simulink model "PID_track"  (R2024b)
settings: Solver=VariableStepAuto  StartTime=0.0  StopTime=t_sim  RelTol=1e-3
values from neighbouring files (symbols this model uses):
  Ax = [0 1; 0 0]    [Main_PID_track.m]
  Ay = [0 1; 0 0]    [Main_PID_track.m]
  b = 0.0245    [Main_PID_track.m]
  Bx = [0 Cx]'    [Main_PID_track.m]
  By = [0 Cy]'    [Main_PID_track.m]
  Cx = m*g*b/(m+J/r^2)/lx    (= 0.943269230769)    [Main_PID_track.m]
  Cy = m*g*b/(m+J/r^2)/ly    (= 1.1445)    [Main_PID_track.m]
  data_sys = [m r g J b lx ly]    [Main_PID_track.m]
  Kb_x = 0.8    [Main_PID_track.m]
  Kb_y = 0.8    [Main_PID_track.m]
  Kd_x = 3    [Main_PID_track.m]
  Kd_y = Kd_x/1.2    (= 2.5)    [Main_PID_track.m]
  Ki_x = 1.5    [Main_PID_track.m]
  Ki_y = Ki_x/1.2    (= 1.25)    [Main_PID_track.m]
  Kp_x = 5    [Main_PID_track.m]
  Kp_y = Kp_x/1.2    (= 4.16666666667)    [Main_PID_track.m]
  lx = 0.182    [Main_PID_track.m]
  ly = 0.150    (= 0.15)    [Main_PID_track.m]
  N_x = 15    [Main_PID_track.m]
  N_y = 15    [Main_PID_track.m]
  ux_lim = 45    [Main_PID_track.m]
  uy_lim = 45    [Main_PID_track.m]
  zx0 = [x0 xp0]'    [Main_PID_track.m]
  zy0 = [y0 yp0]'    [Main_PID_track.m]
undefined symbols (not defined in the file or in its folder): Dx, Dy
libraries: slpidlib x2, simulink x1
settings Model: Creator=nicvi  LastModifiedBy=nicvi

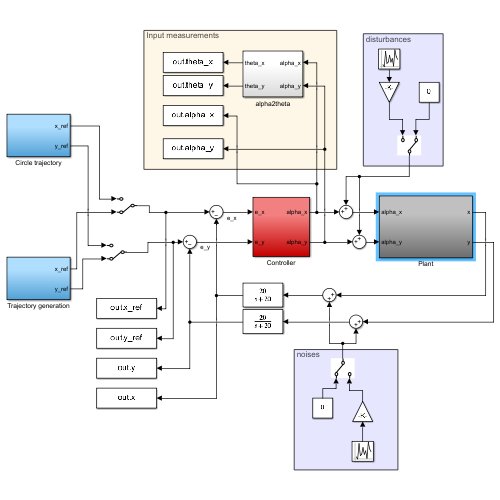
[thumbnail: Simulink's stored preview of the top-level diagram]
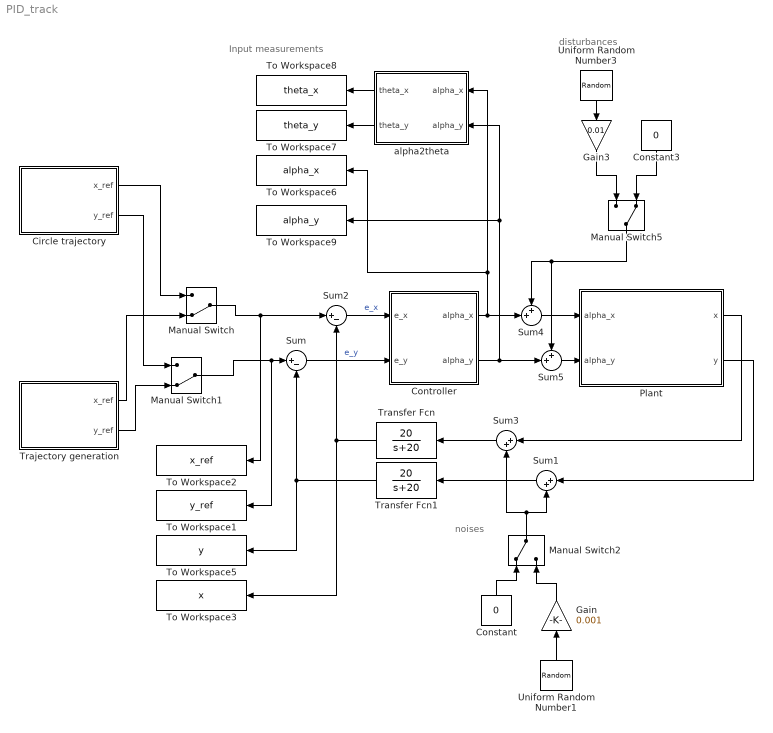
== system PID_track ==
  note: noises
  note: Input measurements
  note: disturbances
  Circle trajectory : Subsystem
  Constant : Constant  Value=0
  Constant3 : Constant  Value=0
  Controller : Subsystem
  Gain : Gain  Gain=0.001
  Gain3 : Gain  Gain=0.01
  Manual Switch : ManualSwitch  CurrentSetting=0
  Manual Switch1 : ManualSwitch  CurrentSetting=0
  Manual Switch2 : ManualSwitch
  Manual Switch5 : ManualSwitch  CurrentSetting=0
  Plant : Subsystem
  Sum : Sum  Inputs=|+-
  Sum1 : Sum  Inputs=|++
  Sum2 : Sum  Inputs=|+-
  Sum3 : Sum  Inputs=|++
  Sum4 : Sum  Inputs=++|
  Sum5 : Sum  Inputs=++|
  To Workspace1 : ToWorkspace  VariableName=y_ref  SampleTime=-1
      settings: Save2DSignal=2-D array (concatenate along first dimension)
  To Workspace2 : ToWorkspace  VariableName=x_ref  SampleTime=-1
      settings: Save2DSignal=2-D array (concatenate along first dimension)
  To Workspace3 : ToWorkspace  VariableName=x  SampleTime=-1
      settings: Save2DSignal=2-D array (concatenate along first dimension)
  To Workspace5 : ToWorkspace  VariableName=y  SampleTime=-1
      settings: Save2DSignal=2-D array (concatenate along first dimension)
  To Workspace6 : ToWorkspace  VariableName=alpha_x  SampleTime=-1
      settings: Save2DSignal=2-D array (concatenate along first dimension)
  To Workspace7 : ToWorkspace  VariableName=theta_y  SampleTime=-1
      settings: Save2DSignal=2-D array (concatenate along first dimension)
  To Workspace8 : ToWorkspace  VariableName=theta_x  SampleTime=-1
      settings: Save2DSignal=2-D array (concatenate along first dimension)
  To Workspace9 : ToWorkspace  VariableName=alpha_y  SampleTime=-1
      settings: Save2DSignal=2-D array (concatenate along first dimension)
  Trajectory generation : Subsystem
  Transfer Fcn : TransferFcn  Numerator=[20]  Denominator=[1 20]
  Transfer Fcn1 : TransferFcn  Numerator=[20]  Denominator=[1 20]
  Uniform Random Number1 : UniformRandomNumber  SampleTime=0.1
  Uniform Random Number3 : UniformRandomNumber  Minimum=5  Maximum=7  SampleTime=0.01
  alpha2theta : Subsystem
  wires:
  Sum2/1 -> Controller/1(e_x)  "e_x"
  Sum/1 -> Controller/2(e_y)  "e_y"
  Controller/1(alpha_x) -> alpha2theta/1(alpha_x), To Workspace6/1, Sum4/2
  Controller/2(alpha_y) -> Sum5/2, alpha2theta/2(alpha_y), To Workspace9/1
  alpha2theta/1(theta_x) -> To Workspace8/1
  alpha2theta/2(theta_y) -> To Workspace7/1
  Plant/2(y) -> Sum1/1
  Plant/1(x) -> Sum3/1
  Circle trajectory/1(x_ref) -> Manual Switch/1
  Manual Switch/1 -> Sum2/1, To Workspace2/1
  Manual Switch1/1 -> To Workspace1/1, Sum/1
  Circle trajectory/2(y_ref) -> Manual Switch1/1
  Trajectory generation/1(x_ref) -> Manual Switch/2
  Trajectory generation/2(y_ref) -> Manual Switch1/2
  Sum1/1 -> Transfer Fcn1/1
  Sum3/1 -> Transfer Fcn/1
  Gain/1 -> Manual Switch2/2
  Manual Switch2/1 -> Sum1/2, Sum3/2
  Uniform Random Number1/1 -> Gain/1
  Transfer Fcn/1 -> Sum2/2, To Workspace3/1
  Transfer Fcn1/1 -> Sum/2, To Workspace5/1
  Constant/1 -> Manual Switch2/1
  Manual Switch5/1 -> Sum4/1, Sum5/1
  Constant3/1 -> Manual Switch5/2
  Uniform Random Number3/1 -> Gain3/1
  Gain3/1 -> Manual Switch5/1
  Sum4/1 -> Plant/1(alpha_x)
  Sum5/1 -> Plant/2(alpha_y)

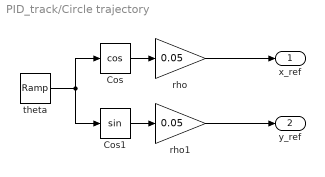
== system PID_track/Circle trajectory ==
  Cos : Trigonometry  Operator=cos
  Cos1 : Trigonometry
  rho : Gain  Gain=0.05
  rho1 : Gain  Gain=0.05
  theta : simulink/Sources/Ramp  slope=2*pi/10  start=0  InitialOutput=0
  x_ref : Outport
  y_ref : Outport  Port=2
  wires:
  theta/1 -> Cos1/1, Cos/1
  Cos/1 -> rho/1
  Cos1/1 -> rho1/1
  rho1/1 -> y_ref/1
  rho/1 -> x_ref/1

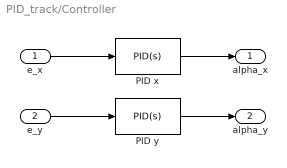
== system PID_track/Controller ==
  e_x : Inport
  e_y : Inport  Port=2
  PID x : slpidlib/PID Controller  Controller=PID  Form=Parallel  TimeDomain=Continuous-time  UseExternalTs=off  SampleTime=-1  IntegratorMethod=Forward Euler  FilterMethod=Forward Euler  ControllerParametersSource=internal  P=Kp_x  I=Ki_x  UseKiTs=off  D=Kd_x  UseExternalDerivativeSource=off  N=N_x  UseFilter=on  TunerSelectOption=Transfer Function Based (PID Tuner App)  InitialConditionSource=internal  InitialConditionForIntegrator=0  InitialConditionForFilter=0  DifferentiatorICPrevScaledInput=0  ExternalReset=none  TrackingMode=off  Kt=1  LimitOutput=on  SatLimitsSource=internal  UpperSaturationLimit=deg2rad(ux_lim)  LowerSaturationLimit=deg2rad(-ux_lim)  LinearizeAsGain=on  AntiWindupMode=back-calculation  Kb=Kb_x  LimitIntegrator=off  UpperIntegratorSaturationLimit=inf  LowerIntegratorSaturationLimit=-inf  POutMin=[]  POutMax=[]  IOutMin=[]  IOutMax=[]  DOutMin=[]  DOutMax=[]  NOutMin=[]  NOutMax=[]  SumOutMin=[]  SumOutMax=[]  SaturationOutMin=[]  SaturationOutMax=[]  PParamMin=[]  PParamMax=[]  IParamMin=[]  IParamMax=[]  DParamMin=[]  DParamMax=[]  NParamMin=[]  NParamMax=[]  KbParamMin=[]  KbParamMax=[]  KtParamMin=[]  KtParamMax=[]  KbOutMin=[]  KbOutMax=[]  KtOutMin=[]  KtOutMax=[]  IntegratorOutMin=[]  IntegratorOutMax=[]  FilterOutMin=[]  FilterOutMax=[]  SumI1OutMin=[]  SumI1OutMax=[]  SumI2OutMin=[]  SumI2OutMax=[]  SumI3OutMin=[]  SumI3OutMax=[]  SumI4OutMin=[]  SumI4OutMax=[]  SumDOutMin=[]  SumDOutMax=[]  DifferentiatorOutMin=[]  DifferentiatorOutMax=[]  FilterDiffOutCoefMin=[]  FilterDiffOutCoefMax=[]  ReciprocalOutMin=[]  ReciprocalOutMax=[]  SumDenOutMin=[]  SumDenOutMax=[]  SumNumOutMin=[]  SumNumOutMax=[]  DivideOutMin=[]  DivideOutMax=[]  UdiffTsProdOutMin=[]  UdiffTsProdOutMax=[]  NTsProdOutMin=[]  NTsProdOutMax=[]  UintegralTsProdOutMin=[]  UintegralTsProdOutMax=[]  UngainTsProdOutMin=[]  UngainTsProdOutMax=[]  ClampingZeroOutDataTypeStr=Inherit: Inherit via back propagation  ClampingZeroOutMin=[]  ClampingZeroOutMax=[]  FilterDenConstantOutDataTypeStr=Inherit: Inherit via back propagation  FilterDenConstantOutMin=[]  FilterDenConstantOutMax=[]  PCopyOutDataTypeStr=Inherit: Inherit via back propagation  PCopyOutMin=[]  PCopyOutMax=[]  NCopyOutDataTypeStr=Inherit: Inherit via back propagation  NCopyOutMin=[]  NCopyOutMax=[]  IntegratorContinuousStateAttributes=''  IntegratorStateMustResolveToSignalObject=off  IntegratorRTWStateStorageClass=Auto  FilterContinuousStateAttributes=''  FilterStateMustResolveToSignalObject=off  FilterRTWStateStorageClass=Auto  ParallelPVariant=InternalParameters  IdealPVariant=Disabled  IVariant=InternalParameters  DVariant=InternalParameters  IntegratorVariant=Continuous  SatVariant=Enabled  AWVariant=BackCalculation  PCopyVariant=Disabled  TRVariant=Disabled  FdbkBlocksVariant=Forward  IdealPFdbkVariant=Disabled  SatFdbkVariant=Disabled  DerivativeFilterVariant=ContFilter  NVariant=InternalParameters  NCopyVariant=Disabled  FilterICVariant=InternalICsFilter  IntegratorICVariant=InternalICs  ExternalResetVariant=Disabled  TRSumVariant=Passthrough  SumFdbkVariant=Disabled  SumVariant=Sum_PID  TsampFilterVariant=InternalTs  TsampNgainVariant=Passthrough  TsampIntegralVariant=Disabled_SignalSpec  ExternalSaturationOutDataTypeStr=Inherit: Same as second input  DerivativeSourceVariant=ErrorSignal  PreIntVariant=InternalPreInt
  PID y : slpidlib/PID Controller  Controller=PID  Form=Parallel  TimeDomain=Continuous-time  UseExternalTs=off  SampleTime=-1  IntegratorMethod=Forward Euler  FilterMethod=Forward Euler  ControllerParametersSource=internal  P=Kp_y  I=Ki_y  UseKiTs=off  D=Kd_y  UseExternalDerivativeSource=off  N=N_y  UseFilter=on  TunerSelectOption=Transfer Function Based (PID Tuner App)  InitialConditionSource=internal  InitialConditionForIntegrator=0  InitialConditionForFilter=0  DifferentiatorICPrevScaledInput=0  ExternalReset=none  TrackingMode=off  Kt=1  LimitOutput=on  SatLimitsSource=internal  UpperSaturationLimit=deg2rad(uy_lim)  LowerSaturationLimit=deg2rad(-uy_lim)  LinearizeAsGain=on  AntiWindupMode=back-calculation  Kb=Kb_y  LimitIntegrator=off  UpperIntegratorSaturationLimit=inf  LowerIntegratorSaturationLimit=-inf  POutMin=[]  POutMax=[]  IOutMin=[]  IOutMax=[]  DOutMin=[]  DOutMax=[]  NOutMin=[]  NOutMax=[]  SumOutMin=[]  SumOutMax=[]  SaturationOutMin=[]  SaturationOutMax=[]  PParamMin=[]  PParamMax=[]  IParamMin=[]  IParamMax=[]  DParamMin=[]  DParamMax=[]  NParamMin=[]  NParamMax=[]  KbParamMin=[]  KbParamMax=[]  KtParamMin=[]  KtParamMax=[]  KbOutMin=[]  KbOutMax=[]  KtOutMin=[]  KtOutMax=[]  IntegratorOutMin=[]  IntegratorOutMax=[]  FilterOutMin=[]  FilterOutMax=[]  SumI1OutMin=[]  SumI1OutMax=[]  SumI2OutMin=[]  SumI2OutMax=[]  SumI3OutMin=[]  SumI3OutMax=[]  SumI4OutMin=[]  SumI4OutMax=[]  SumDOutMin=[]  SumDOutMax=[]  DifferentiatorOutMin=[]  DifferentiatorOutMax=[]  FilterDiffOutCoefMin=[]  FilterDiffOutCoefMax=[]  ReciprocalOutMin=[]  ReciprocalOutMax=[]  SumDenOutMin=[]  SumDenOutMax=[]  SumNumOutMin=[]  SumNumOutMax=[]  DivideOutMin=[]  DivideOutMax=[]  UdiffTsProdOutMin=[]  UdiffTsProdOutMax=[]  NTsProdOutMin=[]  NTsProdOutMax=[]  UintegralTsProdOutMin=[]  UintegralTsProdOutMax=[]  UngainTsProdOutMin=[]  UngainTsProdOutMax=[]  ClampingZeroOutDataTypeStr=Inherit: Inherit via back propagation  ClampingZeroOutMin=[]  ClampingZeroOutMax=[]  FilterDenConstantOutDataTypeStr=Inherit: Inherit via back propagation  FilterDenConstantOutMin=[]  FilterDenConstantOutMax=[]  PCopyOutDataTypeStr=Inherit: Inherit via back propagation  PCopyOutMin=[]  PCopyOutMax=[]  NCopyOutDataTypeStr=Inherit: Inherit via back propagation  NCopyOutMin=[]  NCopyOutMax=[]  IntegratorContinuousStateAttributes=''  IntegratorStateMustResolveToSignalObject=off  IntegratorRTWStateStorageClass=Auto  FilterContinuousStateAttributes=''  FilterStateMustResolveToSignalObject=off  FilterRTWStateStorageClass=Auto  ParallelPVariant=InternalParameters  IdealPVariant=Disabled  IVariant=InternalParameters  DVariant=InternalParameters  IntegratorVariant=Continuous  SatVariant=Enabled  AWVariant=BackCalculation  PCopyVariant=Disabled  TRVariant=Disabled  FdbkBlocksVariant=Forward  IdealPFdbkVariant=Disabled  SatFdbkVariant=Disabled  DerivativeFilterVariant=ContFilter  NVariant=InternalParameters  NCopyVariant=Disabled  FilterICVariant=InternalICsFilter  IntegratorICVariant=InternalICs  ExternalResetVariant=Disabled  TRSumVariant=Passthrough  SumFdbkVariant=Disabled  SumVariant=Sum_PID  TsampFilterVariant=InternalTs  TsampNgainVariant=Passthrough  TsampIntegralVariant=Disabled_SignalSpec  ExternalSaturationOutDataTypeStr=Inherit: Same as second input  DerivativeSourceVariant=ErrorSignal  PreIntVariant=InternalPreInt
  alpha_x : Outport
  alpha_y : Outport  Port=2
  wires:
  PID y/1 -> alpha_y/1
  e_y/1 -> PID y/1
  e_x/1 -> PID x/1
  PID x/1 -> alpha_x/1

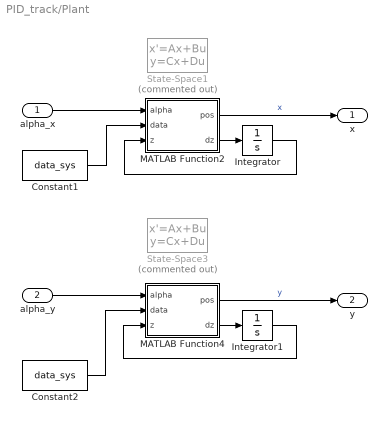
== system PID_track/Plant ==
  alpha_x : Inport
  alpha_y : Inport  Port=2
  Constant1 : Constant  Value=data_sys
  Constant2 : Constant  Value=data_sys
  Integrator : Integrator  InitialCondition=zx0
  Integrator1 : Integrator  InitialCondition=zy0
  MATLAB Function2 : MATLAB Function  TreatAsAtomicUnit=on
  MATLAB Function4 : MATLAB Function  TreatAsAtomicUnit=on
  State-Space1 : StateSpace  Commented=on  A=Ax  B=Bx  C=Cx  D=Dx  InitialCondition=zx0
  State-Space3 : StateSpace  Commented=on  A=Ay  B=By  C=Cy  D=Dy  InitialCondition=zy0
  x : Outport
  y : Outport  Port=2
  wires:
  alpha_y/1 -> MATLAB Function4/1(alpha)
  alpha_x/1 -> MATLAB Function2/1(alpha)
  MATLAB Function2/1(pos) -> x/1  "x"
  Constant1/1 -> MATLAB Function2/2(data)
  MATLAB Function2/2(dz) -> Integrator/1
  Integrator/1 -> MATLAB Function2/3(z)
  MATLAB Function4/2(dz) -> Integrator1/1
  Integrator1/1 -> MATLAB Function4/3(z)
  MATLAB Function4/1(pos) -> y/1  "y"
  Constant2/1 -> MATLAB Function4/2(data)

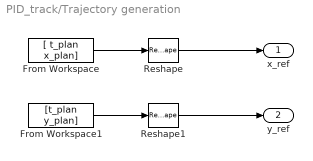
== system PID_track/Trajectory generation ==
  From Workspace : FromWorkspace  VariableName=[ t_plan x_plan]  OutputAfterFinalValue=Holding final value
  From Workspace1 : FromWorkspace  VariableName=[t_plan y_plan]  OutputAfterFinalValue=Holding final value
  Reshape : Reshape  OutputDimensionality=Column vector (2-D)
  Reshape1 : Reshape  OutputDimensionality=Column vector (2-D)
  x_ref : Outport
  y_ref : Outport  Port=2
  wires:
  Reshape/1 -> x_ref/1
  Reshape1/1 -> y_ref/1
  From Workspace/1 -> Reshape/1
  From Workspace1/1 -> Reshape1/1

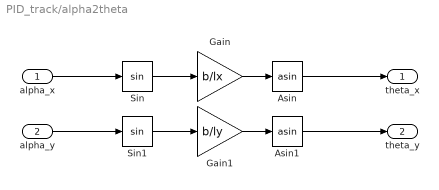
== system PID_track/alpha2theta ==
  alpha_x : Inport
  alpha_y : Inport  Port=2
  Asin : Trigonometry  Operator=asin
  Asin1 : Trigonometry  Operator=asin
  Gain : Gain  Gain=b/lx
  Gain1 : Gain  Gain=b/ly
  Sin : Trigonometry
  Sin1 : Trigonometry
  theta_x : Outport
  theta_y : Outport  Port=2
  wires:
  Gain/1 -> Asin/1
  Sin1/1 -> Gain1/1
  alpha_y/1 -> Sin1/1
  Sin/1 -> Gain/1
  Asin1/1 -> theta_y/1
  Gain1/1 -> Asin1/1
  Asin/1 -> theta_x/1
  alpha_x/1 -> Sin/1

== matlab function PID_track/Plant/MATLAB Function4 ==
  data: pos output; alpha input; dz output; data input; z input
function [pos,dz] = fcn(alpha,data,z)

m=data(1);
r=data(2);
g=data(3);
J=data(4);
b=data(5);
ly=data(7);

Cx=m*g*b/(m+J/r^2)/ly;

dz=zeros(2,1);
dz(1)=z(2);
dz(2)=Cx*sin(alpha);

pos=z(1);

end

== matlab function PID_track/Plant/MATLAB Function2 ==
  data: pos output; alpha input; dz output; data input; z input
function [pos,dz] = fcn(alpha,data,z)

m=data(1);
r=data(2);
g=data(3);
J=data(4);
b=data(5);
lx=data(6);

Cx=m*g*b/(m+J/r^2)/lx;

dz=zeros(2,1);
dz(1)=z(2);
dz(2)=Cx*sin(alpha);

pos=z(1);

end
